simulink model "power_mosconv"  (Simulink 6.0)
settings: Solver=ode23tb  SolverMode=SingleTasking  StartTime=0.0  StopTime=2e-6  RelTol=1e-3
libraries: powerlib x11, simulink x1
settings Model: Creator=patrice  LastModifiedBy=batserve  ExtModeTrigMode=oneshot  ExtModeArmWhenConnect=off  ExtModeAutoUpdateStatusClock=off
settings DataIOCC: LimitDataPoints=off  SignalLoggingName=sigsOut
settings OptimizationCC: BlockReduction=off  BooleanDataType=off
settings DebuggingCC: CheckExecutionContextPreStartOutputMsg=on  CheckExecutionContextRuntimeOutputMsg=on  SolverPrmCheckMsg=none
settings HardwareCC: TargetUnknown=on
settings RTWCC: TemplateMakefile=grt_unix.tmf

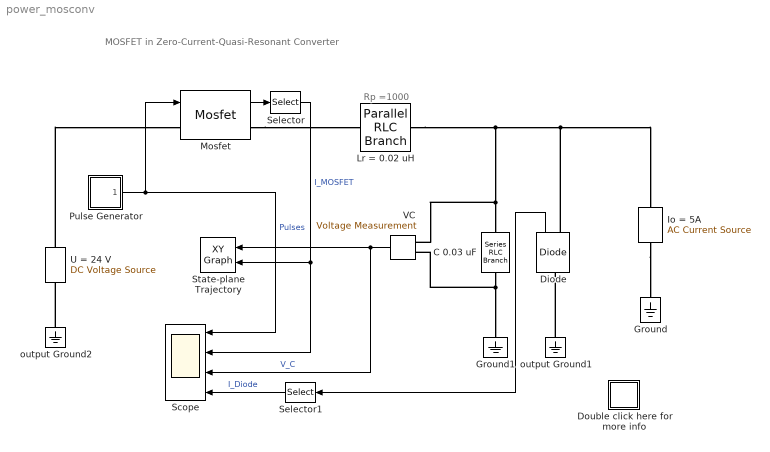
== system power_mosconv ==
  note: MOSFET in Zero-Current-Quasi-Resonant Converter
  note: Rp =1000
  C 0.03 uF : powerlib/Elements/Series RLC Branch  Orientation=down  PhysicalDomain=powersysdomain  SubClassName=unknown  LeftPortType=p1  RightPortType=p1  LConnTagsString=__new0  RConnTagsString=__new0  Resistance=0  Inductance=0  Capacitance=0.03e-6  Measurements=None
  Diode : powerlib/Power Electronics/Diode  Orientation=up  Ron=0.05  Lon=1e-10  Vf=0  IC=5  Rs=inf  Cs=0  Measurements=on
  Double click here for more info : Subsystem
      mask Display: disp('?')
  Ground : powerlib/Elements/Ground  Orientation=down  PhysicalDomain=powersysdomain  SubClassName=unknown  LeftPortType=p1  RightPortType=p1  LConnTagsString=a
  Ground1 : powerlib/Elements/Ground  Orientation=down  PhysicalDomain=powersysdomain  SubClassName=unknown  LeftPortType=p1  RightPortType=p1  LConnTagsString=a
  Io = 5A : powerlib/Electrical Sources/AC Current Source  Orientation=down  Amplitude=5  Phase=90  Frequency=0.01  SampleTime=0  Measurements=None
      settings: AttributesFormatString=\n
  Lr = 0.02 uH : powerlib/Elements/Parallel RLC Branch  PhysicalDomain=powersysdomain  SubClassName=unknown  LeftPortType=p1  RightPortType=p1  LConnTagsString=a  RConnTagsString=__new0  Resistance=1e3  Inductance=0.02e-6  Capacitance=0  Measurements=None
  Mosfet : powerlib/Power Electronics/Mosfet  Ron=5e-3  Lon=1e-9  Rd=5e-5  IC=0  Rs=inf  Cs=0  Measurements=on
      settings: AttributesFormatString=\n
  Pulse Generator : Subsystem  mask(Pulse Generator){period=0.5e-6, duty=20, amplitude=1, start=0}
      mask prompts: period "Period (secs):"; duty "Duty cycle (% of period):"; start "Start time:"
      mask help: Pulse Generator
      mask Help: Pulse generator which ensures pulse transitions are hit. Provides a vector of pulses when the height is entered as a vector.  Unmask to see how it works.
      mask Display: plot(0,0,100,100,[95,90,90,75,75,60,60,45,45,30,30,15,15,5],[25,25,75,75,25,25,75,75,25,25,75,75,25,25]);
  Scope : Scope  NumInputPorts=4
      settings: TimeRange=2e-006  YMin=0~-30~-10~0  YMax=1~40~50~7.5  DataFormat=Array
  Selector : Selector  InputPortWidth=2
  Selector1 : Selector  Orientation=left  InputPortWidth=2
  State-plane Trajectory : simulink/Sinks/XY Graph  Orientation=left  xmin=-5  xmax=50  ymin=-50  ymax=50  st=-1
  U = 24 V : powerlib/Electrical Sources/DC Voltage Source  Description=source block  Orientation=up  Amplitude=24  Measurements=None
      settings: AttributesFormatString=\n
  VC : powerlib/Measurements/Voltage Measurement  Tag=PoWeRsYsTeMmEaSuReMeNt  Orientation=left  PhasorSimulation=off  OutputType=Magnitude  PSBequivalent=0
  output Ground1 : powerlib/Elements/Ground  Orientation=down  PhysicalDomain=powersysdomain  SubClassName=unknown  LeftPortType=p1  RightPortType=p1  LConnTagsString=a
  output Ground2 : powerlib/Elements/Ground  Orientation=down  PhysicalDomain=powersysdomain  SubClassName=unknown  LeftPortType=p1  RightPortType=p1  LConnTagsString=a
  wires:
  Selector1/1 -> Scope/4  "I_Diode"
  Selector/1 -> State-plane Trajectory/2, Scope/2  "I_MOSFET"
  Mosfet/1 -> Selector/1
  Diode/1 -> Selector1/1
  VC/1 -> Scope/3, State-plane Trajectory/1  "V_C"
  Pulse Generator/1(out1) -> Mosfet/1, Scope/1  "Pulses"
  connections:
  Lr = 0.02 uH/RConn1 -- VC/LConn1 -- C 0.03 uF/LConn1 -- Io = 5A/LConn1 -- Diode/RConn1
  C 0.03 uF/RConn1 -- VC/LConn2 -- Ground1/LConn1
  Io = 5A/RConn1 -- Ground/LConn1
  U = 24 V/RConn1 -- Mosfet/LConn1
  output Ground2/LConn1 -- U = 24 V/LConn1
  Mosfet/RConn1 -- Lr = 0.02 uH/LConn1
  output Ground1/LConn1 -- Diode/LConn1

== system power_mosconv/Double click here for more info ==
  note: This  example illustrates use of MOSFET in the Zero-Current
      | Quasi-Resonant Switch (ZCQRS) converter
  note: Circuit Description
  note: The MOSFET is used in a Zero-Current-Quasi-Resonant Switch (ZCQRS) converter topology.
      | In this topology, the device current flows through the resonant tank (Lr, Cr), thus causing zero
      | current turn-off. The load is modeled as an ideal current source (Io). The MOSFET is driven
      | by a 2 MHz pulse train with 20 % duty cycle.
      |
      | Note: In order to avoid cascading two current sources (MOSFET in series with Lr),
      | a parallel resistor Rp of 1000 ohms is connected across Lr.
  note: K. Al-Haddad (Ecole de Technologie Superieure, Montreal)

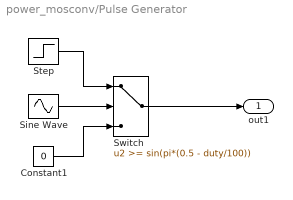
== system power_mosconv/Pulse Generator ==
  Constant1 : Constant  Value=0
  Sine Wave : Sin  Frequency=2*pi./period  Phase=-2*pi*(start./period + duty/200 - 1/4)  SampleTime=0
  Step : Step  Time=start  After=amplitude  SampleTime=0
  Switch : Switch  Threshold=sin(pi*(0.5 - duty/100))  SaturateOnIntegerOverflow=on  InputSameDT=on
  out1 : Outport  InitialOutput=0
  wires:
  Step/1 -> Switch/1
  Constant1/1 -> Switch/3
  Switch/1 -> out1/1
  Sine Wave/1 -> Switch/2
